simulink model "TSTraj"  (R2024a)
settings: Solver=ode8  StartTime=0.0  StopTime=10  FixedStep=0.001  RelTol=1e-3
model workspace (MAT data in the model file):
  q_init_l = Simulink.Parameter
  q_init_l.Value = [0.165747; 0.819274; 1.26369; 0.604148; 1.0515; -0.139217]
  q_init_l.Complexity = 'real'
  q_init_l.Dimensions = [6 1]
  q_init_l.DataType = 'double'
  q_init_r = Simulink.Parameter
  q_init_r.Value = [-0.165747; -0.819274; -1.26369; -0.604148; -1.0515; 0.139217]
  q_init_r.Complexity = 'real'
  q_init_r.Dimensions = [6 1]
  q_init_r.DataType = 'double'
  robot : robotics.RigidBodyTree (value not decoded)
libraries: robotcorelib x2
settings Model: Creator=sung  LastModifiedBy=sung
settings HardwareCC: ProdBitPerLong=64  ProdHWDeviceType=Intel->x86-64 (Linux 64)
settings RTWCC: GenCodeOnly=on  Toolchain=CMake

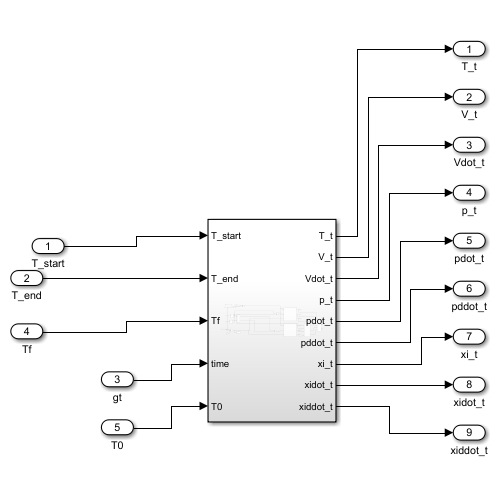
[thumbnail: Simulink's stored preview of the top-level diagram]
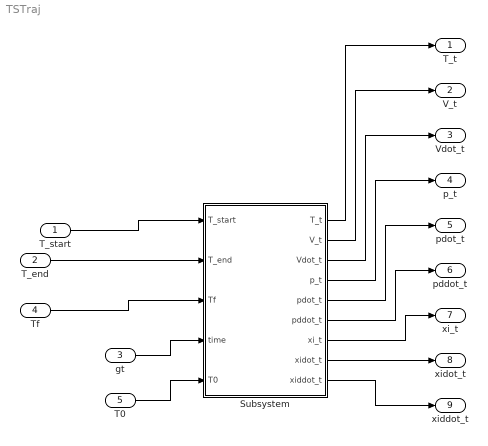
== system TSTraj ==
  T_start : Inport  PortDimensions=[4,4]
  T_end : Inport  Port=2  PortDimensions=[4,4]
  gt : Inport  Port=3
  Tf : Inport  Port=4
  T0 : Inport  Port=5
  Subsystem : Subsystem
  T_t : Outport
  V_t : Outport  Port=2
  Vdot_t : Outport  Port=3
  p_t : Outport  Port=4
  pdot_t : Outport  Port=5
  pddot_t : Outport  Port=6
  xi_t : Outport  Port=7
  xidot_t : Outport  Port=8
  xiddot_t : Outport  Port=9
  wires:
  Subsystem/1(T_t) -> T_t/1
  Subsystem/7(xi_t) -> xi_t/1
  Subsystem/3(Vdot_t) -> Vdot_t/1
  Subsystem/4(p_t) -> p_t/1
  Subsystem/2(V_t) -> V_t/1
  Subsystem/5(pdot_t) -> pdot_t/1
  Subsystem/6(pddot_t) -> pddot_t/1
  Subsystem/8(xidot_t) -> xidot_t/1
  Subsystem/9(xiddot_t) -> xiddot_t/1
  T0/1 -> Subsystem/5(T0)
  Tf/1 -> Subsystem/3(Tf)
  T_end/1 -> Subsystem/2(T_end)
  T_start/1 -> Subsystem/1(T_start)
  gt/1 -> Subsystem/4(time)

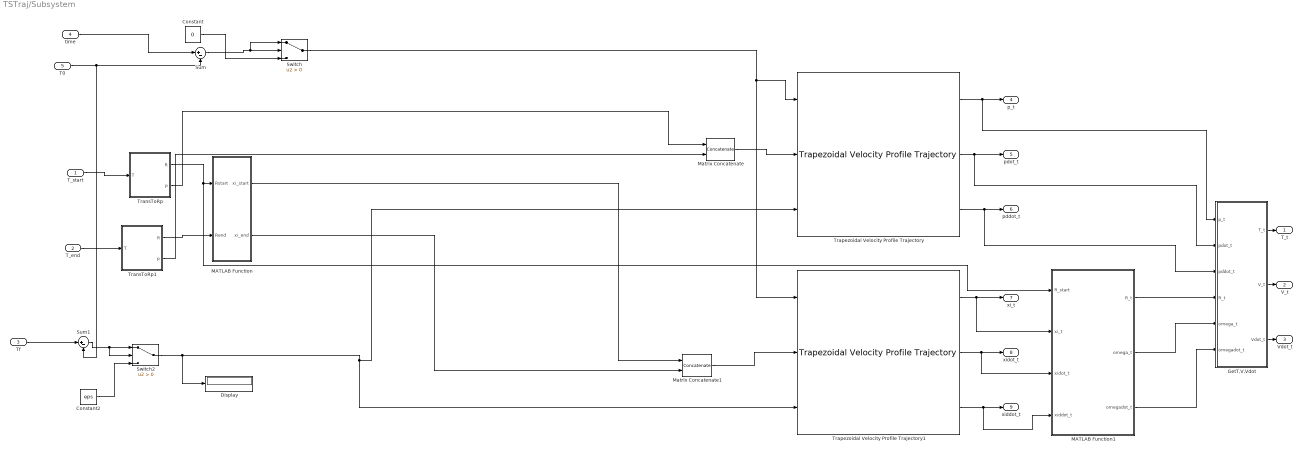
== system TSTraj/Subsystem ==
  T_start : Inport
  T_end : Inport  Port=2
  Tf : Inport  Port=3
  time : Inport  Port=4
  T0 : Inport  Port=5
  Constant : Constant  Value=0
  Constant2 : Constant  Value=eps
  Display : Display
  GetT,V,Vdot : MATLAB Function  TreatAsAtomicUnit=on
  MATLAB Function : MATLAB Function  TreatAsAtomicUnit=on
  MATLAB Function1 : MATLAB Function  TreatAsAtomicUnit=on
  Matrix Concatenate : Concatenate  Mode=Multidimensional array  ConcatenateDimension=2
  Matrix Concatenate1 : Concatenate  Mode=Multidimensional array  ConcatenateDimension=2
  Sum : Sum  Inputs=|+-
  Sum1 : Sum  Inputs=|+-
  Switch : Switch  Criteria=u2 > Threshold  SaturateOnIntegerOverflow=off  InputSameDT=off
  Switch2 : Switch  Criteria=u2 > Threshold  SaturateOnIntegerOverflow=off  InputSameDT=off
  TransToRp : MATLAB Function  TreatAsAtomicUnit=on
  TransToRp1 : MATLAB Function  TreatAsAtomicUnit=on
  Trapezoidal Velocity Profile Trajectory : robotcorelib/Trapezoidal Velocity Profile Trajectory  WaypointSource=External  Waypoints=[ 0, -0.5, -1; 0, 0.5, 1 ]  NumParams=1  Parameter1=End Time  Parameter2=End Time  ParameterSource=External  PeakVelocity=[ 2; 2 ]  Acceleration=[ 1; 2 ]  EndTime=[ 1; 1 ]  AccelTime=[ 1; 2 ]  SimulateUsing=Code generation
  Trapezoidal Velocity Profile Trajectory1 : robotcorelib/Trapezoidal Velocity Profile Trajectory  WaypointSource=External  Waypoints=[ 0, -0.5, -1; 0, 0.5, 1 ]  NumParams=1  Parameter1=End Time  Parameter2=End Time  ParameterSource=External  PeakVelocity=[ 2; 2 ]  Acceleration=[ 1; 2 ]  EndTime=[ 1; 1 ]  AccelTime=[ 1; 2 ]  SimulateUsing=Code generation
  T_t : Outport
  V_t : Outport  Port=2
  Vdot_t : Outport  Port=3
  p_t : Outport  Port=4
  pdot_t : Outport  Port=5
  pddot_t : Outport  Port=6
  xi_t : Outport  Port=7
  xidot_t : Outport  Port=8
  xiddot_t : Outport  Port=9
  wires:
  Trapezoidal Velocity Profile Trajectory/2 -> pdot_t/1, GetT,V,Vdot/2(pdot_t)
  MATLAB Function1/2(omega_t) -> GetT,V,Vdot/5(omega_t)
  MATLAB Function1/1(R_t) -> GetT,V,Vdot/4(R_t)
  TransToRp/1(R) -> MATLAB Function1/1(R_start), MATLAB Function/1(Rstart)
  TransToRp1/2(p) -> Matrix Concatenate/2
  TransToRp/2(p) -> Matrix Concatenate/1
  Trapezoidal Velocity Profile Trajectory1/1 -> xi_t/1, MATLAB Function1/2(xi_t)
  MATLAB Function/1(xi_start) -> Matrix Concatenate1/1
  Trapezoidal Velocity Profile Trajectory1/3 -> xiddot_t/1, MATLAB Function1/4(xiddot_t)
  Matrix Concatenate1/1 -> Trapezoidal Velocity Profile Trajectory1/2
  Trapezoidal Velocity Profile Trajectory1/2 -> xidot_t/1, MATLAB Function1/3(xidot_t)
  MATLAB Function/2(xi_end) -> Matrix Concatenate1/2
  Matrix Concatenate/1 -> Trapezoidal Velocity Profile Trajectory/2
  T_end/1 -> TransToRp1/1(T)
  Trapezoidal Velocity Profile Trajectory/3 -> pddot_t/1, GetT,V,Vdot/3(pddot_t)
  TransToRp1/1(R) -> MATLAB Function/2(Rend)
  MATLAB Function1/3(omegadot_t) -> GetT,V,Vdot/6(omegadot_t)
  Trapezoidal Velocity Profile Trajectory/1 -> p_t/1, GetT,V,Vdot/1(p_t)
  Switch/1 -> Trapezoidal Velocity Profile Trajectory1/1, Trapezoidal Velocity Profile Trajectory/1
  GetT,V,Vdot/3(Vdot_t) -> Vdot_t/1
  GetT,V,Vdot/1(T_t) -> T_t/1
  GetT,V,Vdot/2(V_t) -> V_t/1
  T_start/1 -> TransToRp/1(T)
  time/1 -> Sum/1
  T0/1 -> Sum/2, Sum1/2
  Sum/1 -> Switch/1, Switch/2
  Switch2/1 -> Display/1, Trapezoidal Velocity Profile Trajectory1/3, Trapezoidal Velocity Profile Trajectory/3
  Tf/1 -> Sum1/1
  Sum1/1 -> Switch2/2, Switch2/1
  Constant2/1 -> Switch2/3
  Constant/1 -> Switch/3

== matlab function TSTraj/Subsystem/GetT,V,Vdot ==
  data: p_t input; T_t output; pdot_t input; pddot_t input; R_t input; omega_t input; omegadot_t input; V_t output; Vdot_t output
function [T_t,V_t,Vdot_t] = getTVVdot(p_t,pdot_t,pddot_t,R_t,omega_t,omegadot_t)

T_t = RpToTrans(R_t,p_t);
V_t = [R_t'*pdot_t;omega_t];
Rdot_t = (R_t*VecToso3(omega_t))';
Vdot_t = [Rdot_t'*pdot_t+R_t'*pddot_t;omegadot_t];

== matlab function TSTraj/Subsystem/MATLAB Function ==
  data: Rstart input; xi_start output; Rend input; xi_end output
function [xi_start,xi_end] = fcn(Rstart,Rend)

xi_start = zeros(3,1);
xi_end = zeros(3,1);

xi_end = so3ToVec(MatrixLog3((Rstart)'*Rend));

== matlab function TSTraj/Subsystem/MATLAB Function1 ==
  data: R_start input; R_t output; xi_t input; omega_t output; omegadot_t output; xidot_t input; xiddot_t input
function [R_t,omega_t,omegadot_t] = ExpCoordinateToSO3(R_start,xi_t,xidot_t,xiddot_t)
R_t = eye(3);
omega_t = zeros(3,1);
omegadot_t = zeros(3,1);


R_t = R_start*MatrixExp3(VecToso3(xi_t));
omega_t = dexp3(-xi_t)*xidot_t;
omegadot_t = dexp3(-xi_t)*xiddot_t+ ddexp3(-xi_t,-xidot_t)*xidot_t;

== matlab function TSTraj/Subsystem/TransToRp ==
  data: T input; R output; p output
function [R,p] = TransToRp(T)

[R,p] = TransToRp(T);

== matlab function TSTraj/Subsystem/TransToRp1 ==
  data: T input; R output; p output
function [R,p] = TransToRp(T)

[R,p] = TransToRp(T);
